simulink model "sim_model"  (Simulink 10.1)
settings: Solver=FixedStepAuto  StartTime=0  StopTime=10  FixedStep=0.01  RelTol=0.001  EnableMultiTasking=on
libraries: fmu_me_lib x1
settings Model: Creator=Tin Rabuzin  LastModifiedBy=meagh
settings DataIOCC: LimitDataPoints=on  OutputSaveName=simout  OutputOption=SpecifiedOutputTimes  OutputTimes=[0:0.01:10]
settings OptimizationCC: ExpressionDepthLimit=2147483647
settings DebuggingCC: SolverPrmCheckMsg=warning  StateNameClashWarn=warning
settings GRTTargetCC: CombineOutputUpdateFcns=on  GRTInterface=off

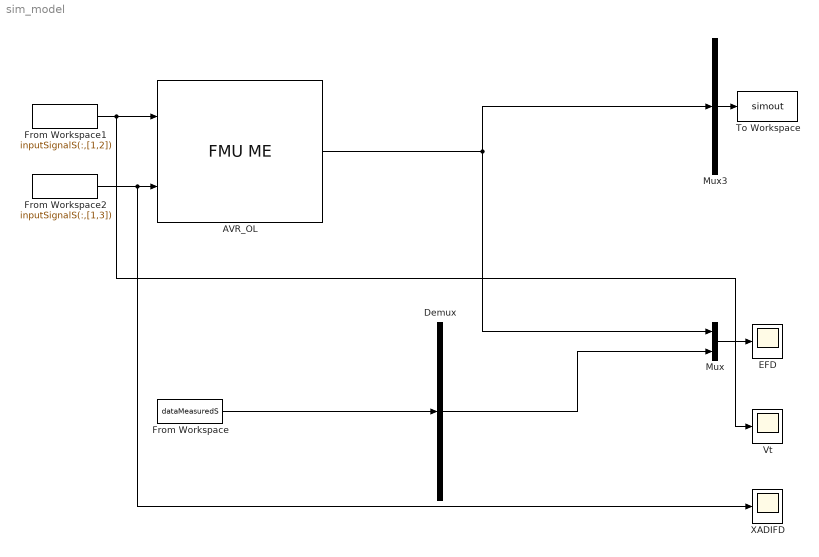
== system sim_model ==
  AVR_OL : fmu_me_lib/FMU ME  Description=Simulates an FMU for Model Exchange 1.0 or Model Exchange 2.0.  dummy=0
  Demux : Demux  Outputs=1
  EFD : Scope
  From Workspace : FromWorkspace  VariableName=dataMeasuredS
  From Workspace1 : FromWorkspace  VariableName=inputSignalS(:,[1,2])
  From Workspace2 : FromWorkspace  VariableName=inputSignalS(:,[1,3])
  Mux : Mux  Inputs=2
  Mux3 : Mux  Inputs=1
  To Workspace : ToWorkspace  VariableName=simout  SaveFormat=Structure With Time  SampleTime=-1
  Vt : Scope
  XADIFD : Scope
  wires:
  From Workspace/1 -> Demux/1
  Mux3/1 -> To Workspace/1
  Mux/1 -> EFD/1
  AVR_OL/1 -> Mux3/1, Mux/1
  From Workspace1/1 -> Vt/1, AVR_OL/1
  From Workspace2/1 -> XADIFD/1, AVR_OL/2
  Demux/1 -> Mux/2
